simulink model "quadModel"  (Simulink 8.4)
settings: Solver=ode45  StartTime=0.0  StopTime=10.0  RelTol=1e-3
settings Model: Creator=Alexey  LastModifiedBy=Dejan
settings DataIOCC: SignalLoggingSaveFormat=Dataset
settings OptimizationCC: InlineParams=on
settings DebuggingCC: FcnCallInpInsideContextMsg=EnableAllAsError
settings GRTTargetCC: CombineOutputUpdateFcns=on  GRTInterface=off

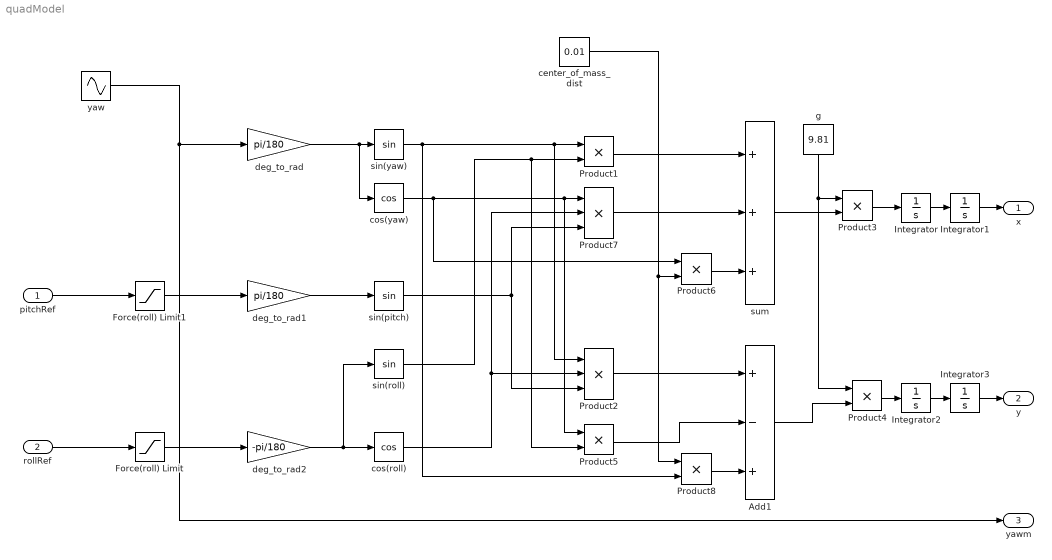
== system quadModel ==
  pitchRef : Inport
  rollRef : Inport  Port=2
  Add1 : Sum  Inputs=+-+
  Force(roll) Limit : Saturate  UpperLimit=30  LowerLimit=-30
  Force(roll) Limit1 : Saturate  UpperLimit=30  LowerLimit=-30
  Integrator : Integrator
  Integrator1 : Integrator  InitialCondition=0.75
  Integrator2 : Integrator
  Integrator3 : Integrator  InitialCondition=0.75
  Product{1,3..6,8} (6 alike) : Product  RndMeth=Zero
  Product2 : Product  Inputs=3  RndMeth=Zero
  Product7 : Product  Inputs=3  RndMeth=Zero
  center_of_mass_dist : Constant  Value=0.01
  cos(roll) : Trigonometry  Operator=cos
  cos(yaw) : Trigonometry  Operator=cos
  deg_to_rad : Gain  Gain=pi/180
  deg_to_rad1 : Gain  Gain=pi/180
  deg_to_rad2 : Gain  Gain=-pi/180
  g : Constant  Value=9.81
  sin(pitch) : Trigonometry
  sin(roll) : Trigonometry
  sin(yaw) : Trigonometry
  sum : Sum  Inputs=+++
  yaw : Sin  Amplitude=0  Frequency=0.25  SampleTime=0
  x : Outport
  y : Outport  Port=2
  yawm : Outport  Port=3
  wires:
  sin(yaw)/1 -> Product8/2, Product2/1, Product1/1
  cos(yaw)/1 -> Product6/1, Product5/1, Product7/1
  yaw/1 -> yawm/1, deg_to_rad/1
  deg_to_rad/1 -> cos(yaw)/1, sin(yaw)/1
  deg_to_rad1/1 -> sin(pitch)/1
  sin(pitch)/1 -> Product2/3, Product7/3
  deg_to_rad2/1 -> sin(roll)/1, cos(roll)/1
  cos(roll)/1 -> Product7/2, Product2/2
  sin(roll)/1 -> Product5/2, Product1/2
  Product1/1 -> sum/1
  Product7/1 -> sum/2
  Product5/1 -> Add1/2
  Product2/1 -> Add1/1
  g/1 -> Product4/1, Product3/1
  sum/1 -> Product3/2
  Add1/1 -> Product4/2
  Product3/1 -> Integrator/1
  Integrator1/1 -> x/1
  Integrator/1 -> Integrator1/1
  Product4/1 -> Integrator2/1
  Integrator2/1 -> Integrator3/1
  Integrator3/1 -> y/1
  Force(roll) Limit1/1 -> deg_to_rad1/1
  pitchRef/1 -> Force(roll) Limit1/1
  Force(roll) Limit/1 -> deg_to_rad2/1
  rollRef/1 -> Force(roll) Limit/1
  Product6/1 -> sum/3
  center_of_mass_dist/1 -> Product8/1, Product6/2
  Product8/1 -> Add1/3
